simulink model "L1E2"  (R2019b)
settings: Solver=VariableStepAuto  StartTime=0.0  StopTime=100  RelTol=1e-3
model workspace (MAT data in the model file):
  m = Simulink.Parameter
  m.DataType = 'auto'
  m.Dimensions = [0 0]
settings Model: Creator=Callum  LastModifiedBy=Callum
settings DataIOCC: ReturnWorkspaceOutputs=off

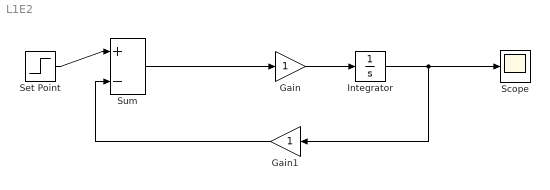
== system L1E2 ==
  Gain : Gain
  Gain1 : Gain
  Integrator : Integrator
  Scope : Scope
  Set Point : Step  Time=10  After=10  SampleTime=0
  Sum : Sum  Inputs=|+-
  wires:
  Integrator/1 -> Gain1/1, Scope/1
  Gain/1 -> Integrator/1
  Set Point/1 -> Sum/1
  Gain1/1 -> Sum/2
  Sum/1 -> Gain/1
